simulink model "model_of_system_theta_DC"  (R2021a)
settings: Solver=VariableStepAuto  StartTime=0.0  StopTime=86400  RelTol=1e-3
libraries: fl_lib x88, nesl_utility x28, ee_lib x18, SimscapeFluids_lib x6, simulink x1
(part 1 of 2)
settings Model: OrderedModelArguments=off  Creator=SINA  LastModifiedBy=SINA
settings SolverCC: ZeroCrossAlgorithm=Adaptive
settings DebuggingCC: IgnoredZcDiagnostic=none

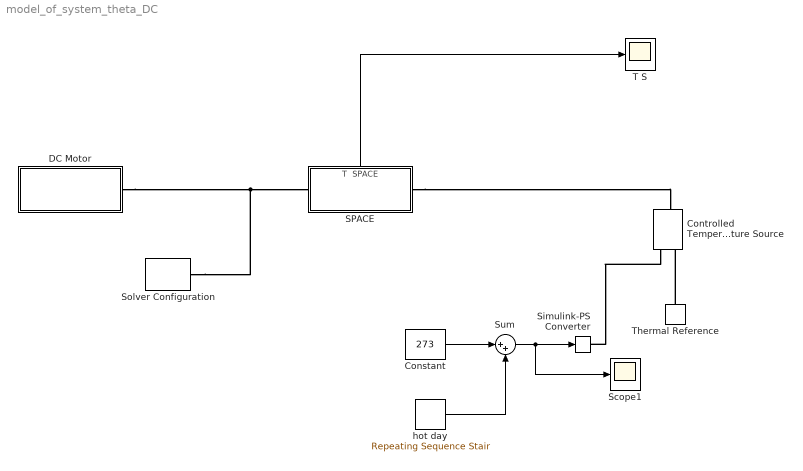
== system model_of_system_theta_DC ==
  Constant : Constant  Value=273
  Controlled Temperature Source : fl_lib/Thermal/Thermal Sources/Controlled Temperature Source
  DC Motor : Subsystem
  "SPACE " : Subsystem
      settings: PortSchema="{\"entries\":[{\"content\":{\"sides\":[{\"content\":{\"connectorIds\":[\"LConn1\"]},\"type\":\"ConnectorPlacement.EquallySpacedRectSide\",\"uuid\":\"d6720360-fd14-4102-8920-24b0f3e87daf\"},{\"content\":{\"connectorIds\":[\"RConn1\"],\"side\":\"RIGHT\"},\"type\":\"ConnectorPlacement.EquallySpacedRectSide\",\"uuid\":\"8de063fd-0e95-49b0-b131-452f09033aa1\"},{\"content\":{\"connectorIds\":[\"Out1\"],\"side\":\"TOP\"},\"type\":\"ConnectorPlacement.EquallySpacedRectSide\",\"uuid\":\"37599775-f873-4ff0-934d-fcf325c50c65\"}]},\"type\":\"ConnectorPlacement.EquallySpacedConnector\",\"uuid\":\"8fae0317-fc8f-430a-90e7-4ae7dd04f39d\"}],\"packageUris\":[\"http://schema.mathworks.com/mf0/Connector/R2020b\"],\"version\":\"1.0\"}"
  Scope1 : Scope
  Simulink-PS Converter : nesl_utility/Simulink-PS Converter  PhysicalDomain=network_engine_domain  SubClassName=ps_input  LeftPortType=input  RightPortType=output  PseudoPeriodic=off  Frequencies=[]  NoiseDistribution=none  NoiseParameters=[]  Unit=K  AffineConversion=off  FilteringAndDerivatives=provide  SimscapeFilterOrder=1  InputFilterTimeConstant=0.001  UdotUserProvided=0
      settings: SourceProductBaseCode=PW,SS
  Solver Configuration : nesl_utility/Solver Configuration  PhysicalDomain=network_engine_domain  SubClassName=solver  LeftPortType=input  RightPortType=generic  Tones=[]  Harmonics=[]  SimulateNoise=off  Profile=off  UseLocalSampling=off  EnableSwitchedLinearOptims=on  FrequencyDomain=off  UseCCode=off  RelTol=0.001  AbsTol=1e-06  MinStep=1e-09  ToWorkspace=off  RevertToSquareIcSolve=off  NumHomotopyIterations=100  PhasorMode=off  PhasorModeNumHarmonics=1  DoDC=off  ResidualTolerance=1e-09  UseLocalSolver=off  LocalSolverChoice=NE_BACKWARD_EULER_ADVANCER  LocalSolverSampleTime=0.001  DoFixedCost=off  MaxNonlinIter=3  MaxModeIter=2  ComputeImpulses=off  ImpulseIterations=2  LinearAlgebra=auto  EquationFormulation=NE_TIME_EF  DelaysMemoryBudget=1024  AutomaticFiltering=on  FilteringTimeConstant=0.001  PartitionStorageMethod=AS_NEEDED  PartitionMemoryBudget=1024  PartitionMethod=ROBUST
      settings: SourceProductBaseCode=PW,SS
  Sum : Sum  Inputs=|++
  T S : Scope
  Thermal Reference : fl_lib/Thermal/Thermal Elements/Thermal Reference
  "hot day " : simulink/Sources/Repeating Sequence Stair  OutValues=|  tsamp=600  OutMin=[]  OutMax=[]  OutDataTypeStr=double  OutputDataTypeScalingMode=double  OutDataType=fixdt(0,8)  ConRadixGroup=Best Precision: Vector-wise  OutScaling=2^-12
      | [19.7
      | 19.8
      | 19.9
      | 19.6
      | 19.3
      | 19
      | 18.9
      | 18.8
      | 18.7
      | 18.6
      | 18.4
      | 18.3
      | 18.4
      | 18.5
      | 18.6
      | 18.6
      | 18.7
      | 18.5
      | 18.5
      | 18.5
      | 18.7
      | 18.9
      | 19.1
      | 19.6
      | 20
      | 20.3
      | 20.7
      | 20.9
      | 20.8
      | 20.7
      | 20.8
      | 21.4
      | 22.1
      | 22.7
      | 23
      | 23.7
      | 24.3
      | 25.2
      | 25.8
      | 25.8
      | 26.2
      | 26.5
      | 26.7
      | 26.7
      | 26.7
      | 27.8
      | 28.2
      | 28.4
      | 29.1
      | 29.5
      | 30.2
      | 30.8
      | 30.8
      | 31.2
      | 31.5
      | 31.4
      | 31.3
      | 31.3
      | 31.2
      | 31.4
      | 31.5
      | 31.5
      | 31.6
      | 31.5
      | 31.6
      | 31.3
      | 31.2
      | 31.2
      | 31.2
      | 31.9
      | 31.7
      | 31.4
      | 31.3
      | 31.6
      | 32.4
      | 32.3
      | 31.9
      | 32
      | 32.1
      | 32.1
      | 32.2
      | 32
      | 32.1
      | 32.1
      | 32.3
      | 32.3
      | 31.9
      | 31.4
      | 31.5
      | 31.5
      | 31
      | 30.6
      | 29.7
      | 28.9
      | 28.4
      | 28.1
      | 27.4
      | 26.6
      | 25.6
      | 24.5
      | 23.7
      | 22.9
      | 22.5
      | 22.2
      | 22
      | 21.9
      | 21.7
      | 21.4
      | 21.2
      | 21.1
      | 20.9
      | 20.9
      | 20.8
      | 20.7
      | 20.6
      | 20.2
      | 20
      | 19.9
      | 19.9
      | 19.9
      | 19.8
      | 19.6
      | 19.4
      | 19.1
      | 19
      | 19
      | 19
      | 18.9
      | 18.8
      | 18.7
      | 18.7
      | 18.3
      | 18
      | 17.7
      | 17.5
      | 17.5
      | 17.4
      | 17.3
      | 17.1
      | 17
      | 16.9
      | 16.8
      | 16.6
      | 16.5
      | 16.5
      | ]
  wires:
  Constant/1 -> Sum/1
  Sum/1 -> Scope1/1, Simulink-PS Converter/1
  "hot day "/1 -> Sum/2
  "SPACE "/1(T  SPACE) -> T S/1
  connections:
  Thermal Reference/LConn1 -- Controlled Temperature Source/RConn2
  Controlled Temperature Source/RConn1 -- Simulink-PS Converter/RConn1
  "SPACE "/RConn1 -- Controlled Temperature Source/LConn1
  DC Motor/LConn1 -- Solver Configuration/RConn1 -- "SPACE "/LConn1

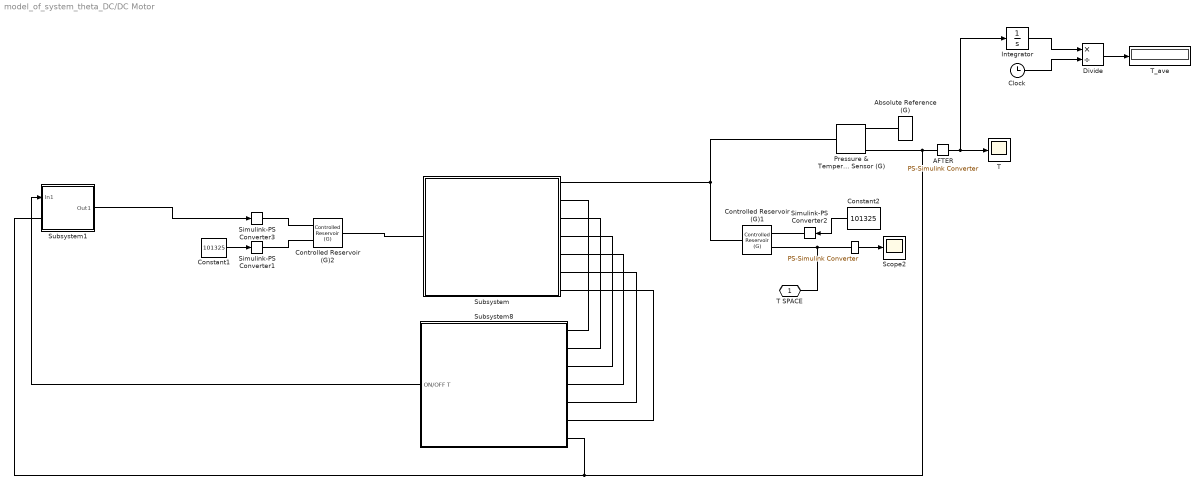
== system model_of_system_theta_DC/DC Motor ==
  " " : nesl_utility/PS-Simulink Converter  PhysicalDomain=network_engine_domain  SubClassName=ps_output  LeftPortType=input  RightPortType=output  PseudoPeriodic=off  Frequencies=[]  Unit=K  AffineConversion=off
      settings: SourceProductBaseCode=PW,SS
  AFTER : nesl_utility/PS-Simulink Converter  PhysicalDomain=network_engine_domain  SubClassName=ps_output  LeftPortType=input  RightPortType=output  PseudoPeriodic=off  Frequencies=[]  Unit=K  AffineConversion=off
      settings: SourceProductBaseCode=PW,SS
  Absolute Reference (G) : fl_lib/Gas/Elements/Absolute Reference (G)
      settings: SourceProductBaseCode=SS  InternalSimscapePortConfiguration="{\"Bottom\":[],\"Left\":[{\"id\":\"A\",\"label\":\"\",\"type\":\"foundation.gas.gas\"}],\"Right\":[],\"Top\":[]}"
  Clock : Clock
  Constant1 : Constant  Value=101325
  Constant2 : Constant  Value=101325
  Controlled Reservoir (G)1 : fl_lib/Gas/Elements/Controlled Reservoir (G)  area_A=25 m^2
      settings: SourceProductBaseCode=SS  InternalSimscapePortConfiguration="{\"Bottom\":[],\"Left\":[{\"id\":\"A\",\"label\":\"A\",\"type\":\"foundation.gas.gas\"}],\"Right\":[{\"id\":\"T_in\",\"label\":\"T\",\"type\":\"input\"},{\"id\":\"p_in\",\"label\":\"P\",\"type\":\"input\"}],\"Top\":[]}"
  Controlled Reservoir (G)2 : fl_lib/Gas/Elements/Controlled Reservoir (G)  area_A=40 m^2
      settings: SourceProductBaseCode=SS  InternalSimscapePortConfiguration="{\"Bottom\":[],\"Left\":[{\"id\":\"A\",\"label\":\"A\",\"type\":\"foundation.gas.gas\"}],\"Right\":[{\"id\":\"T_in\",\"label\":\"T\",\"type\":\"input\"},{\"id\":\"p_in\",\"label\":\"P\",\"type\":\"input\"}],\"Top\":[]}"
  Divide : Product  Inputs=*/
  Integrator : Integrator
  Pressure & Temperature Sensor (G) : fl_lib/Gas/Sensors/Pressure & Temperature Sensor (G)
      settings: SourceProductBaseCode=SS  InternalSimscapePortConfiguration="{\"Bottom\":[],\"Left\":[{\"id\":\"A\",\"label\":\"A\",\"type\":\"foundation.gas.gas\"}],\"Right\":[{\"id\":\"B\",\"label\":\"B\",\"type\":\"foundation.gas.gas\"},{\"id\":\"P\",\"label\":\"P\",\"type\":\"output\"},{\"id\":\"T\",\"label\":\"T\",\"type\":\"output\"}],\"Top\":[]}"
  Scope2 : Scope
  Simulink-PS Converter1 : nesl_utility/Simulink-PS Converter  PhysicalDomain=network_engine_domain  SubClassName=ps_input  LeftPortType=input  RightPortType=output  PseudoPeriodic=off  Frequencies=[]  NoiseDistribution=none  NoiseParameters=[]  Unit=Pa  AffineConversion=off  FilteringAndDerivatives=provide  SimscapeFilterOrder=1  InputFilterTimeConstant=0.001  UdotUserProvided=0
      settings: SourceProductBaseCode=PW,SS
  Simulink-PS Converter2 : nesl_utility/Simulink-PS Converter  PhysicalDomain=network_engine_domain  SubClassName=ps_input  LeftPortType=input  RightPortType=output  PseudoPeriodic=off  Frequencies=[]  NoiseDistribution=none  NoiseParameters=[]  Unit=Pa  AffineConversion=off  FilteringAndDerivatives=provide  SimscapeFilterOrder=1  InputFilterTimeConstant=0.001  UdotUserProvided=0
      settings: SourceProductBaseCode=PW,SS
  Simulink-PS Converter3 : nesl_utility/Simulink-PS Converter  PhysicalDomain=network_engine_domain  SubClassName=ps_input  LeftPortType=input  RightPortType=output  PseudoPeriodic=off  Frequencies=[]  NoiseDistribution=none  NoiseParameters=[]  Unit=K  AffineConversion=off  FilteringAndDerivatives=provide  SimscapeFilterOrder=1  InputFilterTimeConstant=0.001  UdotUserProvided=0
      settings: SourceProductBaseCode=PW,SS
  Subsystem : Subsystem
  Subsystem1 : Subsystem
  Subsystem8 : Subsystem
  T : Scope
  T_ave : Display
  "T SPACE " : PMIOPort  Side=Left
  wires:
  Constant1/1 -> Simulink-PS Converter1/1
  " "/1 -> Scope2/1
  Constant2/1 -> Simulink-PS Converter2/1
  Clock/1 -> Divide/2
  Divide/1 -> T_ave/1
  Integrator/1 -> Divide/1
  AFTER/1 -> T/1, Integrator/1
  Subsystem8/1(ON/OFF T) -> Subsystem1/1(In1)
  Subsystem1/1(Out1) -> Simulink-PS Converter3/1
  connections:
  " "/LConn1 -- "T SPACE "/RConn1 -- Controlled Reservoir (G)1/RConn1
  Simulink-PS Converter3/RConn1 -- Controlled Reservoir (G)2/RConn1
  Simulink-PS Converter1/RConn1 -- Controlled Reservoir (G)2/RConn2
  Simulink-PS Converter2/RConn1 -- Controlled Reservoir (G)1/RConn2
  Absolute Reference (G)/LConn1 -- Pressure & Temperature Sensor (G)/RConn1
  Pressure & Temperature Sensor (G)/LConn1 -- Controlled Reservoir (G)1/LConn1 -- Subsystem/RConn1
  Subsystem/LConn1 -- Controlled Reservoir (G)2/LConn1
  Subsystem8/LConn1 -- Subsystem/RConn2
  Subsystem8/LConn2 -- Subsystem/RConn3
  Subsystem8/LConn3 -- Subsystem/RConn4
  Subsystem8/LConn4 -- Subsystem/RConn5
  Subsystem8/LConn5 -- Subsystem/RConn6
  Subsystem/RConn7 -- Subsystem8/LConn6
  AFTER/LConn1 -- Subsystem1/LConn1 -- Subsystem8/LConn7 -- Pressure & Temperature Sensor (G)/RConn3

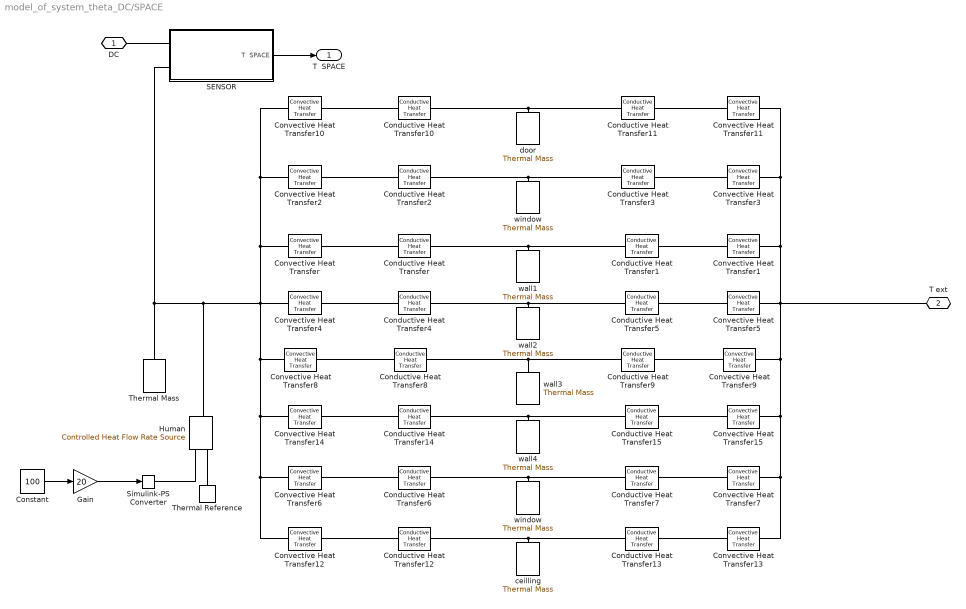
== system model_of_system_theta_DC/SPACE  ==
  " ceilling" : fl_lib/Thermal/Thermal Elements/Thermal Mass  mass=6400 kg  sp_heat=835 J/kg/K  T_specify=on  T_priority=None  T=295 K  T_nominal_specify=off  T_nominal_unit=K  T_nominal_value=1  Q_specify=off  Q_priority=None  Q=0 W  Q_nominal_specify=off  Q_nominal_unit=W  Q_nominal_value=1
  " window" : fl_lib/Thermal/Thermal Elements/Thermal Mass  mass=162 kg  sp_heat=840 J/kg/K  T_specify=on  T_priority=None  T=295 K  T_nominal_specify=off  T_nominal_unit=K  T_nominal_value=1  Q_specify=off  Q_priority=None  Q=0 W  Q_nominal_specify=off  Q_nominal_unit=W  Q_nominal_value=1
  Conductive Heat Transfer{,1,4..5} (4 alike) : fl_lib/Thermal/Thermal Elements/Conductive Heat Transfer  area=320 m^2  thickness=.2 m  th_cond=.038 W/(m*K)  T_specify=off  T_priority=None  T=0 K  T_nominal_specify=off  T_nominal_unit=K  T_nominal_value=1  Q_specify=off  Q_priority=None  Q=0 W  Q_nominal_specify=off  Q_nominal_unit=W  Q_nominal_value=1
  Conductive Heat Transfer10 : fl_lib/Thermal/Thermal Elements/Conductive Heat Transfer  area=7 m^2  thickness=0.04 m  th_cond=.78 W/(m*K)  T_specify=off  T_priority=None  T=0 K  T_nominal_specify=off  T_nominal_unit=K  T_nominal_value=1  Q_specify=off  Q_priority=None  Q=0 W  Q_nominal_specify=off  Q_nominal_unit=W  Q_nominal_value=1
  Conductive Heat Transfer11 : fl_lib/Thermal/Thermal Elements/Conductive Heat Transfer  area=7 m^2  thickness=.04 m  th_cond=.78 W/(m*K)  T_specify=off  T_priority=None  T=0 K  T_nominal_specify=off  T_nominal_unit=K  T_nominal_value=1  Q_specify=off  Q_priority=None  Q=0 W  Q_nominal_specify=off  Q_nominal_unit=W  Q_nominal_value=1
  Conductive Heat Transfer12 : fl_lib/Thermal/Thermal Elements/Conductive Heat Transfer  area=1000 m^2  thickness=0.1 m  th_cond=.038 W/(m*K)  T_specify=off  T_priority=None  T=0 K  T_nominal_specify=off  T_nominal_unit=K  T_nominal_value=1  Q_specify=off  Q_priority=None  Q=0 W  Q_nominal_specify=off  Q_nominal_unit=W  Q_nominal_value=1
  Conductive Heat Transfer13 : fl_lib/Thermal/Thermal Elements/Conductive Heat Transfer  area=1e-4 m^2  thickness=0.1 m  th_cond=.038 W/(m*K)  T_specify=off  T_priority=None  T=0 K  T_nominal_specify=off  T_nominal_unit=K  T_nominal_value=1  Q_specify=off  Q_priority=None  Q=0 W  Q_nominal_specify=off  Q_nominal_unit=W  Q_nominal_value=1
  Conductive Heat Transfer{8..9,14..15} (4 alike) : fl_lib/Thermal/Thermal Elements/Conductive Heat Transfer  area=150 m^2  thickness=.2 m  th_cond=.038 W/(m*K)  T_specify=off  T_priority=None  T=0 K  T_nominal_specify=off  T_nominal_unit=K  T_nominal_value=1  Q_specify=off  Q_priority=None  Q=0 W  Q_nominal_specify=off  Q_nominal_unit=W  Q_nominal_value=1
  Conductive Heat Transfer{2..3,6..7} (4 alike) : fl_lib/Thermal/Thermal Elements/Conductive Heat Transfer  area=6 m^2  thickness=.01 m  th_cond=.78 W/(m*K)  T_specify=off  T_priority=None  T=0 K  T_nominal_specify=off  T_nominal_unit=K  T_nominal_value=1  Q_specify=off  Q_priority=None  Q=0 W  Q_nominal_specify=off  Q_nominal_unit=W  Q_nominal_value=1
  Constant : Constant  Value=100
  Convective Heat Transfer{,1,4..5} (4 alike) : fl_lib/Thermal/Thermal Elements/Convective Heat Transfer  area=320 m^2  heat_tr_coeff=24 W/(m^2 * K)  T_specify=off  T_priority=None  T=0 K  T_nominal_specify=off  T_nominal_unit=K  T_nominal_value=1  Q_specify=off  Q_priority=None  Q=0 W  Q_nominal_specify=off  Q_nominal_unit=W  Q_nominal_value=1
  Convective Heat Transfer10 : fl_lib/Thermal/Thermal Elements/Convective Heat Transfer  area=7 m^2  heat_tr_coeff=26 W/(m^2 * K)  T_specify=off  T_priority=None  T=0 K  T_nominal_specify=off  T_nominal_unit=K  T_nominal_value=1  Q_specify=off  Q_priority=None  Q=0 W  Q_nominal_specify=off  Q_nominal_unit=W  Q_nominal_value=1
  Convective Heat Transfer11 : fl_lib/Thermal/Thermal Elements/Convective Heat Transfer  area=7 m^2  heat_tr_coeff=26 W/(m^2 * K)  T_specify=off  T_priority=None  T=0 K  T_nominal_specify=off  T_nominal_unit=K  T_nominal_value=1  Q_specify=off  Q_priority=None  Q=0 W  Q_nominal_specify=off  Q_nominal_unit=W  Q_nominal_value=1
  Convective Heat Transfer12 : fl_lib/Thermal/Thermal Elements/Convective Heat Transfer  area=1000 m^2  heat_tr_coeff=12 W/(m^2 * K)  T_specify=off  T_priority=None  T=0 K  T_nominal_specify=off  T_nominal_unit=K  T_nominal_value=1  Q_specify=off  Q_priority=None  Q=0 W  Q_nominal_specify=off  Q_nominal_unit=W  Q_nominal_value=1
  Convective Heat Transfer13 : fl_lib/Thermal/Thermal Elements/Convective Heat Transfer  area=1000 m^2  heat_tr_coeff=12 W/(m^2 * K)  T_specify=off  T_priority=None  T=0 K  T_nominal_specify=off  T_nominal_unit=K  T_nominal_value=1  Q_specify=off  Q_priority=None  Q=0 W  Q_nominal_specify=off  Q_nominal_unit=W  Q_nominal_value=1
  Convective Heat Transfer{8..9,14..15} (4 alike) : fl_lib/Thermal/Thermal Elements/Convective Heat Transfer  area=150 m^2  heat_tr_coeff=24 W/(m^2 * K)  T_specify=off  T_priority=None  T=0 K  T_nominal_specify=off  T_nominal_unit=K  T_nominal_value=1  Q_specify=off  Q_priority=None  Q=0 W  Q_nominal_specify=off  Q_nominal_unit=W  Q_nominal_value=1
  Convective Heat Transfer{2..3,6..7} (4 alike) : fl_lib/Thermal/Thermal Elements/Convective Heat Transfer  area=6 m^2  heat_tr_coeff=25 W/(m^2 * K)  T_specify=off  T_priority=None  T=0 K  T_nominal_specify=off  T_nominal_unit=K  T_nominal_value=1  Q_specify=off  Q_priority=None  Q=0 W  Q_nominal_specify=off  Q_nominal_unit=W  Q_nominal_value=1
  Gain : Gain  Gain=20
  Human : fl_lib/Thermal/Thermal Sources/Controlled Heat Flow Rate Source
  SENSOR : Subsystem
  Simulink-PS Converter : nesl_utility/Simulink-PS Converter  PhysicalDomain=network_engine_domain  SubClassName=ps_input  LeftPortType=input  RightPortType=output  PseudoPeriodic=off  Frequencies=[]  NoiseDistribution=none  NoiseParameters=[]  Unit=J/s  AffineConversion=off  FilteringAndDerivatives=provide  SimscapeFilterOrder=1  InputFilterTimeConstant=0.001  UdotUserProvided=0
      settings: SourceProductBaseCode=PW,SS
  Thermal Mass : fl_lib/Thermal/Thermal Elements/Thermal Mass  mass=10200 kg  sp_heat=1 J/kg/K  T_specify=on  T_priority=High  T=295 K  T_nominal_specify=off  T_nominal_unit=K  T_nominal_value=1  Q_specify=off  Q_priority=None  Q=0 W  Q_nominal_specify=off  Q_nominal_unit=W  Q_nominal_value=1
  Thermal Reference : fl_lib/Thermal/Thermal Elements/Thermal Reference
  door : fl_lib/Thermal/Thermal Elements/Thermal Mass  mass=165 kg  sp_heat=840 J/kg/K  T_specify=on  T_priority=None  T=295 K  T_nominal_specify=off  T_nominal_unit=K  T_nominal_value=1  Q_specify=off  Q_priority=None  Q=0 W  Q_nominal_specify=off  Q_nominal_unit=W  Q_nominal_value=1
  wall1 : fl_lib/Thermal/Thermal Elements/Thermal Mass  mass=122880 kg  sp_heat=835 J/kg/K  T_specify=on  T_priority=None  T=295 K  T_nominal_specify=off  T_nominal_unit=K  T_nominal_value=1  Q_specify=off  Q_priority=None  Q=0 W  Q_nominal_specify=off  Q_nominal_unit=W  Q_nominal_value=1
  wall2 : fl_lib/Thermal/Thermal Elements/Thermal Mass  mass=122880 kg  sp_heat=835 J/kg/K  T_specify=on  T_priority=None  T=295 K  T_nominal_specify=off  T_nominal_unit=K  T_nominal_value=1  Q_specify=off  Q_priority=None  Q=0 W  Q_nominal_specify=off  Q_nominal_unit=W  Q_nominal_value=1
  wall3 : fl_lib/Thermal/Thermal Elements/Thermal Mass  mass=57600 kg  sp_heat=835 J/kg/K  T_specify=on  T_priority=None  T=295 K  T_nominal_specify=off  T_nominal_unit=K  T_nominal_value=1  Q_specify=off  Q_priority=None  Q=0 W  Q_nominal_specify=off  Q_nominal_unit=W  Q_nominal_value=1
  wall4 : fl_lib/Thermal/Thermal Elements/Thermal Mass  mass=57600 kg  sp_heat=835 J/kg/K  T_specify=on  T_priority=None  T=295 K  T_nominal_specify=off  T_nominal_unit=K  T_nominal_value=1  Q_specify=off  Q_priority=None  Q=0 W  Q_nominal_specify=off  Q_nominal_unit=W  Q_nominal_value=1
  window : fl_lib/Thermal/Thermal Elements/Thermal Mass  mass=162 kg  sp_heat=840 J/kg/K  T_specify=on  T_priority=None  T=295 K  T_nominal_specify=off  T_nominal_unit=K  T_nominal_value=1  Q_specify=off  Q_priority=None  Q=0 W  Q_nominal_specify=off  Q_nominal_unit=W  Q_nominal_value=1
  DC : PMIOPort  Side=Left
  T ext : PMIOPort  Port=2  Side=Right
  T  SPACE : Outport  SampleTime=1
  wires:
  SENSOR/1(T  SPACE) -> T  SPACE/1
  Constant/1 -> Gain/1
  Gain/1 -> Simulink-PS Converter/1
  connections:
  Convective Heat Transfer/RConn1 -- Conductive Heat Transfer/LConn1
  Conductive Heat Transfer/RConn1 -- Conductive Heat Transfer1/LConn1 -- wall1/LConn1
  Convective Heat Transfer1/LConn1 -- Conductive Heat Transfer1/RConn1
  Conductive Heat Transfer3/LConn1 -- Conductive Heat Transfer2/RConn1 -- window/LConn1
  Convective Heat Transfer2/RConn1 -- Conductive Heat Transfer2/LConn1
  Convective Heat Transfer3/LConn1 -- Conductive Heat Transfer3/RConn1
  Conductive Heat Transfer5/LConn1 -- Conductive Heat Transfer4/RConn1 -- wall2/LConn1
  Convective Heat Transfer4/RConn1 -- Conductive Heat Transfer4/LConn1
  Convective Heat Transfer5/LConn1 -- Conductive Heat Transfer5/RConn1
  Conductive Heat Transfer6/RConn1 -- Conductive Heat Transfer7/LConn1 -- " window"/LConn1
  Convective Heat Transfer7/LConn1 -- Conductive Heat Transfer7/RConn1
  Convective Heat Transfer6/RConn1 -- Conductive Heat Transfer6/LConn1
  Convective Heat Transfer2/LConn1 -- Convective Heat Transfer10/LConn1 -- Human/LConn1 -- SENSOR/LConn2 -- Thermal Mass/LConn1 -- Convective Heat Transfer4/LConn1 -- Convective Heat Transfer14/LConn1 -- Convective Heat Transfer12/LConn1 -- Convective Heat Transfer6/LConn1 -- Convective Heat Transfer8/LConn1 -- Convective Heat Transfer/LConn1
  Conductive Heat Transfer8/RConn1 -- Conductive Heat Transfer9/LConn1 -- wall3/LConn1
  Convective Heat Transfer9/LConn1 -- Conductive Heat Transfer9/RConn1
  Convective Heat Transfer8/RConn1 -- Conductive Heat Transfer8/LConn1
  Conductive Heat Transfer10/RConn1 -- Conductive Heat Transfer11/LConn1 -- door/LConn1
  Convective Heat Transfer11/LConn1 -- Conductive Heat Transfer11/RConn1
  Convective Heat Transfer10/RConn1 -- Conductive Heat Transfer10/LConn1
  Convective Heat Transfer11/RConn1 -- Convective Heat Transfer5/RConn1 -- Convective Heat Transfer15/RConn1 -- Convective Heat Transfer13/RConn1 -- Convective Heat Transfer7/RConn1 -- Convective Heat Transfer9/RConn1 -- T ext/RConn1 -- Convective Heat Transfer1/RConn1 -- Convective Heat Transfer3/RConn1
  Conductive Heat Transfer13/LConn1 -- " ceilling"/LConn1 -- Conductive Heat Transfer12/RConn1
  Convective Heat Transfer13/LConn1 -- Conductive Heat Transfer13/RConn1
  Convective Heat Transfer12/RConn1 -- Conductive Heat Transfer12/LConn1
  DC/RConn1 -- SENSOR/LConn1
  Conductive Heat Transfer14/RConn1 -- Conductive Heat Transfer15/LConn1 -- wall4/LConn1
  Convective Heat Transfer15/LConn1 -- Conductive Heat Transfer15/RConn1
  Convective Heat Transfer14/RConn1 -- Conductive Heat Transfer14/LConn1
  Human/RConn1 -- Simulink-PS Converter/RConn1
  Thermal Reference/LConn1 -- Human/RConn2

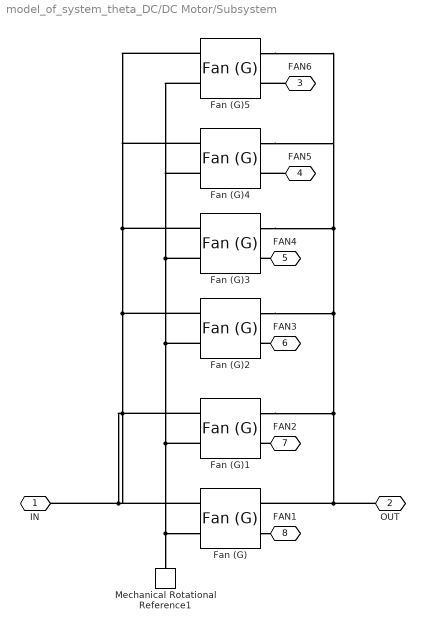
== system model_of_system_theta_DC/DC Motor/Subsystem ==
  Fan (G){,1..4} (5 alike) : SimscapeFluids_lib/Gas/Turbomachinery/Fan (G)  fan_spec=fluids.gas.enum.fan_spec.table2D_dp_dpmax_omega  mech_orientation=simscape.enum.posneg.positive  flow_rate_1D_TLU=[4.7, 5.2, 5.7, 6.1, 6.6] m^3/s  Dp_1D_TLU=[1120, 995.36, 870.94, 746.52, 622.1] Pa  eta_1D_TLU=[.1, .2, .25, .15, .1]  rho_ref_1D=1.2 kg/m^3  omega_ref_1D=910 rpm  omega_Dp_TLU=[2000,2500,3000] rpm  flow_rate_Dp_TLU=[.2, .3, .4, .5] m^3/s  Dp_TLU=[675, 650, 560, 420; 830, 800, 695, 520; 1008, 966, 840, 630; 1200, 1150, 1000, 750; 1370, 1300, 1250, 1000] Pa  eta_Dp_TLU=ones(3,20).*0.3  omega_flow_TLU=[1800, 2000, 2400, 2800, 3000] rpm  Dp_flow_TLU=[1 / 8, 1 / 4, 3 / 8, 1 / 2] * 3386.4 Pa  flow_rate_TLU=[.3282, .2965, .2556, .1973; .8254, .71, .5876, .4545; 1.2018, 1.0829, .9083, .7034; 1.5065, 1.4098, 1.2722, .9844; 1.8368, 1.7507, 1.6055, 1.2417] m^3/s  eta_flow_TLU=[.22, .23, .25, .24; .38, .39, .4, .34; .58, .6, .62, .6; .81, .82, .84, .8; .88, .91, .95, .9]  omega_DpMax_TLU=[2000,2500,3000] rpm  DpMax_TLU=[16.100000000000000,24.500000000000000,34.800000000000000] Pa  omega_flow_TLU_=[2000,2500,3000] rpm  Dp_DpMax_TLU=[0,0.0526315789473684,0.105263157894737,0.157894736842105,0.210526315789474,0.263157894736842,0.315789473684211,0.368421052631579,0.421052631578947,0.473684210526316,0.526315789473684,0.578947368421053,0.631578947368421,0.684210526315790,0.736842105263158,0.789473684210526,0.842105263157895,0.894736842105263,0.947368421052632,1]  flow_rate_TLU_=[16.1273000000000,15.8178000000000,15.0681000000000,14.2018000000000,12.9433000000000,11.3991000000000,9.67790000000000,8.08610000000000,7.01870000000000,6.30920000000000,5.93980000000000,5.97320000000000,5.86980000000000,5.71970000000000,5.52780000000000,5.20060000000000,4.55740000000000,3.42180000000000,1.76410000000000,0.000100000000000000;24.5333000000000,24.3970000000000,23.8165000000000,23.1737000000000,21.5953000000000,19.0999000000000,16.6546000000000,14.3745000000000,12.7327000000000,11.8387000000000,11.3795000000000,11.0625000000000,10.7728000000000,10.4860000000000,10.0474000000000,9.13940000000000,7.85700000000000,5.63250000000000,3.16660000000000,0.000100000000000000;34.8365000000000,34.2986000000000,33.4330000000000,32.3142000000000,30.4522000000000,27.7361000000000,24.3880000000000,21.6723000000000,19.7551000000000,18.4534000000000,17.3506000000000,16.6400000000000,15.8701000000000,14.8205000000000,13.6975000000000,11.7356000000000,9.67960000000000,6.82460000000000,3.51230000000000,0.000100000000000000] lpm  eta_flow_TLU_=ones(3,20).*0.3  rho_ref_2D=1.2 kg/m^3  omega_threshold=1 rpm  area_A=2 m^2  area_B=2 m^2
      settings: SourceProductBaseCode=SH  InternalSimscapePortConfiguration="{\"Bottom\":[],\"Left\":[{\"id\":\"A\",\"label\":\"A\",\"type\":\"foundation.gas.gas\"},{\"id\":\"C\",\"label\":\"C\",\"type\":\"foundation.mechanical.rotational.rotational\"}],\"Right\":[{\"id\":\"B\",\"label\":\"B\",\"type\":\"foundation.gas.gas\"},{\"id\":\"R\",\"label\":\"R\",\"type\":\"foundation.mechanical.rotational.rotational\"}],\"Top\":[]}"
  Fan (G)5 : SimscapeFluids_lib/Gas/Turbomachinery/Fan (G)  fan_spec=fluids.gas.enum.fan_spec.table2D_dp_dpmax_omega  mech_orientation=simscape.enum.posneg.positive  flow_rate_1D_TLU=[4.7, 5.2, 5.7, 6.1, 6.6] m^3/s  Dp_1D_TLU=[1120, 995.36, 870.94, 746.52, 622.1] Pa  eta_1D_TLU=[.1, .2, .25, .15, .1]  rho_ref_1D=1.2 kg/m^3  omega_ref_1D=910 rpm  omega_Dp_TLU=[2000,2500,3000] rpm  flow_rate_Dp_TLU=[.2, .3, .4, .5] m^3/s  Dp_TLU=[675, 650, 560, 420; 830, 800, 695, 520; 1008, 966, 840, 630; 1200, 1150, 1000, 750; 1370, 1300, 1250, 1000] Pa  eta_Dp_TLU=ones(3,20).*0.3  omega_flow_TLU=[1800, 2000, 2400, 2800, 3000] rpm  Dp_flow_TLU=[1 / 8, 1 / 4, 3 / 8, 1 / 2] * 3386.4 Pa  flow_rate_TLU=[.3282, .2965, .2556, .1973; .8254, .71, .5876, .4545; 1.2018, 1.0829, .9083, .7034; 1.5065, 1.4098, 1.2722, .9844; 1.8368, 1.7507, 1.6055, 1.2417] m^3/s  eta_flow_TLU=[.22, .23, .25, .24; .38, .39, .4, .34; .58, .6, .62, .6; .81, .82, .84, .8; .88, .91, .95, .9]  omega_DpMax_TLU=[2000,2500,3000] rpm  DpMax_TLU=[16.100000000000000,24.500000000000000,34.800000000000000] Pa  omega_flow_TLU_=[2000,2500,3000] rad/s  Dp_DpMax_TLU=[0,0.0526315789473684,0.105263157894737,0.157894736842105,0.210526315789474,0.263157894736842,0.315789473684211,0.368421052631579,0.421052631578947,0.473684210526316,0.526315789473684,0.578947368421053,0.631578947368421,0.684210526315790,0.736842105263158,0.789473684210526,0.842105263157895,0.894736842105263,0.947368421052632,1]  flow_rate_TLU_=[16.1273000000000,15.8178000000000,15.0681000000000,14.2018000000000,12.9433000000000,11.3991000000000,9.67790000000000,8.08610000000000,7.01870000000000,6.30920000000000,5.93980000000000,5.97320000000000,5.86980000000000,5.71970000000000,5.52780000000000,5.20060000000000,4.55740000000000,3.42180000000000,1.76410000000000,0.000100000000000000;24.5333000000000,24.3970000000000,23.8165000000000,23.1737000000000,21.5953000000000,19.0999000000000,16.6546000000000,14.3745000000000,12.7327000000000,11.8387000000000,11.3795000000000,11.0625000000000,10.7728000000000,10.4860000000000,10.0474000000000,9.13940000000000,7.85700000000000,5.63250000000000,3.16660000000000,0.000100000000000000;34.8365000000000,34.2986000000000,33.4330000000000,32.3142000000000,30.4522000000000,27.7361000000000,24.3880000000000,21.6723000000000,19.7551000000000,18.4534000000000,17.3506000000000,16.6400000000000,15.8701000000000,14.8205000000000,13.6975000000000,11.7356000000000,9.67960000000000,6.82460000000000,3.51230000000000,0.000100000000000000] lpm  eta_flow_TLU_=ones(3,20).*0.3  rho_ref_2D=1.2 kg/m^3  omega_threshold=1 rpm  area_A=2 m^2  area_B=2 m^2
      settings: SourceProductBaseCode=SH  InternalSimscapePortConfiguration="{\"Bottom\":[],\"Left\":[{\"id\":\"A\",\"label\":\"A\",\"type\":\"foundation.gas.gas\"},{\"id\":\"C\",\"label\":\"C\",\"type\":\"foundation.mechanical.rotational.rotational\"}],\"Right\":[{\"id\":\"B\",\"label\":\"B\",\"type\":\"foundation.gas.gas\"},{\"id\":\"R\",\"label\":\"R\",\"type\":\"foundation.mechanical.rotational.rotational\"}],\"Top\":[]}"
  Mechanical Rotational Reference1 : fl_lib/Mechanical/Rotational Elements/Mechanical Rotational Reference
  IN : PMIOPort  Side=Left
  OUT : PMIOPort  Port=2  Side=Right
  FAN6 : PMIOPort  Port=3  Side=Right
  FAN5 : PMIOPort  Port=4  Side=Right
  FAN4 : PMIOPort  Port=5  Side=Right
  FAN3 : PMIOPort  Port=6  Side=Right
  FAN2 : PMIOPort  Port=7  Side=Right
  FAN1 : PMIOPort  Port=8  Side=Right
  connections:
  Fan (G)1/RConn1 -- Fan (G)2/RConn1 -- Fan (G)5/RConn1 -- Fan (G)4/RConn1 -- Fan (G)3/RConn1 -- Fan (G)/RConn1 -- OUT/RConn1
  FAN4/RConn1 -- Fan (G)3/RConn2
  Fan (G)/LConn1 -- Fan (G)5/LConn1 -- Fan (G)4/LConn1 -- Fan (G)3/LConn1 -- Fan (G)2/LConn1 -- Fan (G)1/LConn1 -- IN/RConn1
  Fan (G)5/LConn2 -- Fan (G)4/LConn2 -- Fan (G)3/LConn2 -- Fan (G)2/LConn2 -- Fan (G)1/LConn2 -- Mechanical Rotational Reference1/LConn1 -- Fan (G)/LConn2
  FAN2/RConn1 -- Fan (G)1/RConn2
  FAN5/RConn1 -- Fan (G)4/RConn2
  FAN6/RConn1 -- Fan (G)5/RConn2
  FAN3/RConn1 -- Fan (G)2/RConn2
  Fan (G)/RConn2 -- FAN1/RConn1

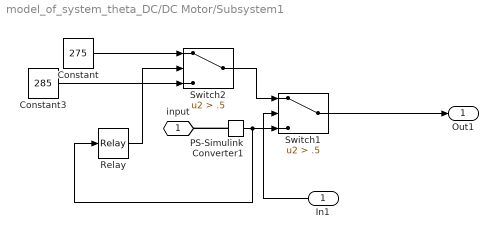
== system model_of_system_theta_DC/DC Motor/Subsystem1 ==
  In1 : Inport
  Constant : Constant  Value=275
  Constant3 : Constant  Value=285
  PS-Simulink Converter1 : nesl_utility/PS-Simulink Converter  PhysicalDomain=network_engine_domain  SubClassName=ps_output  LeftPortType=input  RightPortType=output  PseudoPeriodic=off  Frequencies=[]  Unit=inherit  AffineConversion=off
      settings: SourceProductBaseCode=PW,SS
  Relay : Relay  OnSwitchValue=299  OffSwitchValue=296
  Switch1 : Switch  Criteria=u2 > Threshold  Threshold=.5
  Switch2 : Switch  Criteria=u2 > Threshold  Threshold=.5
  input : PMIOPort  Side=Left
  Out1 : Outport
  wires:
  In1/1 -> Switch1/2
  Switch2/1 -> Switch1/1
  PS-Simulink Converter1/1 -> Relay/1, Switch1/3
  Relay/1 -> Switch2/2
  Constant/1 -> Switch2/1
  Constant3/1 -> Switch2/3
  Switch1/1 -> Out1/1
  connections:
  PS-Simulink Converter1/LConn1 -- input/RConn1

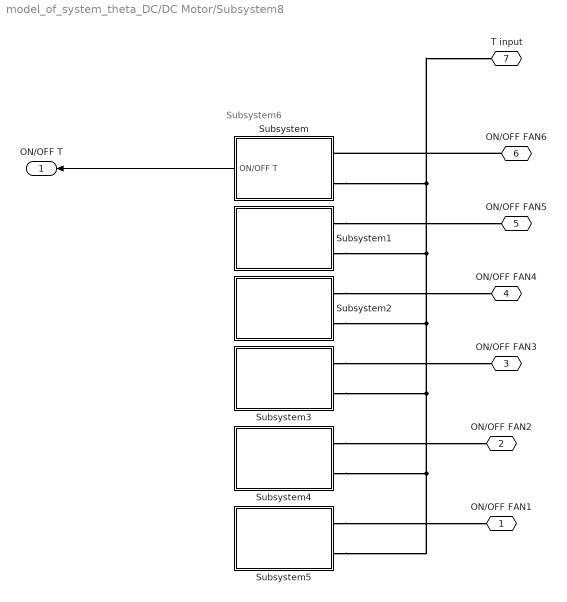
== system model_of_system_theta_DC/DC Motor/Subsystem8 ==
  note: Subsystem6
  Subsystem : Subsystem
  Subsystem1 : Subsystem
  Subsystem2 : Subsystem
  Subsystem3 : Subsystem
  Subsystem4 : Subsystem
  Subsystem5 : Subsystem
  ON/OFF FAN1 : PMIOPort  Side=Left
  ON/OFF FAN2 : PMIOPort  Port=2  Side=Left
  ON/OFF FAN3 : PMIOPort  Port=3  Side=Left
  ON/OFF FAN4 : PMIOPort  Port=4  Side=Left
  ON/OFF FAN5 : PMIOPort  Port=5  Side=Left
  ON/OFF FAN6 : PMIOPort  Port=6  Side=Left
  T input : PMIOPort  Port=7  Side=Left
  ON/OFF T : Outport
  wires:
  Subsystem/1(ON/OFF T) -> ON/OFF T/1
  connections:
  Subsystem1/LConn1 -- ON/OFF FAN5/RConn1
  Subsystem2/LConn1 -- ON/OFF FAN4/RConn1
  Subsystem3/LConn1 -- ON/OFF FAN3/RConn1
  Subsystem4/LConn1 -- ON/OFF FAN2/RConn1
  Subsystem5/LConn1 -- ON/OFF FAN1/RConn1
  Subsystem5/LConn2 -- Subsystem2/LConn2 -- T input/RConn1 -- Subsystem/LConn2 -- Subsystem1/LConn2 -- Subsystem3/LConn2 -- Subsystem4/LConn2
  ON/OFF FAN6/RConn1 -- Subsystem/LConn1

== system model_of_system_theta_DC/SPACE /SENSOR ==
  PS-Simulink Converter : nesl_utility/PS-Simulink Converter  PhysicalDomain=network_engine_domain  SubClassName=ps_output  LeftPortType=input  RightPortType=output  PseudoPeriodic=off  Frequencies=[]  Unit=K  AffineConversion=off
      settings: SourceProductBaseCode=PW,SS
  Scope : Scope
  Temperature Sensor : fl_lib/Thermal/Thermal Sensors/Temperature Sensor
  Thermal Reference1 : fl_lib/Thermal/Thermal Elements/Thermal Reference
  FAN : PMIOPort  Side=Left
  Conn2 : PMIOPort  Port=2  Side=Left
  T  SPACE : Outport  SampleTime=1
  wires:
  PS-Simulink Converter/1 -> T  SPACE/1, Scope/1
  connections:
  Temperature Sensor/RConn2 -- FAN/RConn1 -- PS-Simulink Converter/LConn1
  Temperature Sensor/LConn1 -- Conn2/RConn1
  Thermal Reference1/LConn1 -- Temperature Sensor/RConn1

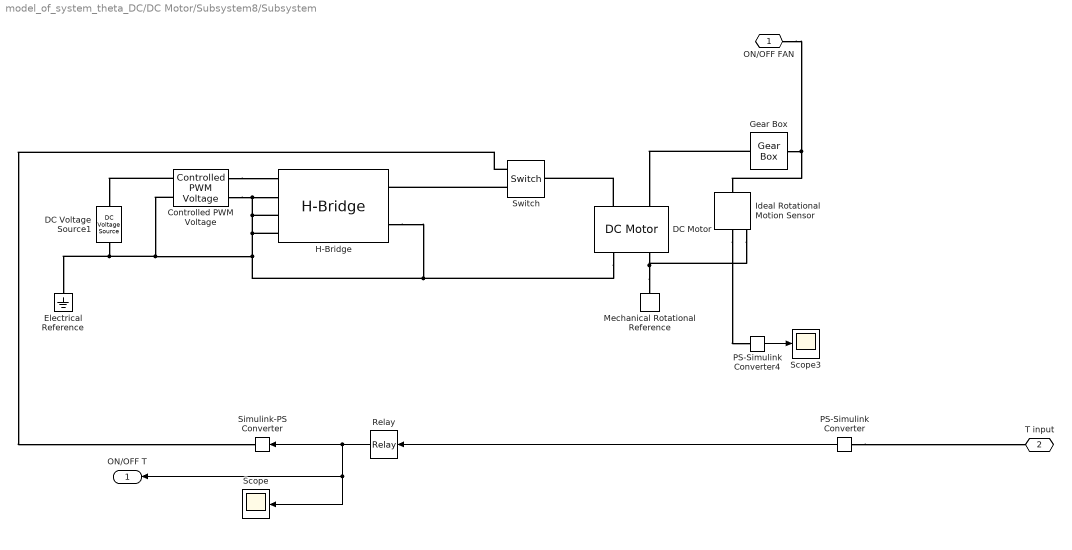
== system model_of_system_theta_DC/DC Motor/Subsystem8/Subsystem ==
  Controlled PWM Voltage : ee_lib/Integrated Circuits/Controlled PWM Voltage  F=4000 Hz  TD=0 s  pulse_width_offset=0 s  pulse_min=0 s  Vmin=0 V  Vmax=5 V  Vm=5 V  pwm_or_av=2  event_type=1  sample_time=1e-6 s  u_min=0  u_max=1
  DC Motor : ee_lib/Electromechanical/Brushed Motors/DC Motor  field_option=ee.enum.field_option.pm  Rf=100 Ohm  Lf=1 H  Laf=0.15 H  If0=0 A  parameterization=ee.enum.dcparam_option.load_speed  Ra=3.9 Ohm  La=.01 H  emf_or_torque=ee.enum.emf_or_torque.kv  Kv=0.072e-3 V/rpm  Ki=6.876e-4 N*m/A  T_stall=0.24e-3 N*m  w_max=4000 rpm  w_rated=1000 rpm  P_rated=10 W  V_rated=12 V  J=0.0002 kg*m^2  lam_param=ee.enum.lam_param.damping  lam=0.5e-5 N*m/(rad/s)  i_noload=0 A  V_i_noload=1.5 V  speed0=0 rpm  enable_fault_armature=ee.enum.faults.faultEnable.no  rev_faulted=1 / 3  G_faulted_armature=1e-5 S  fault_trigger_armature=ee.enum.faults.faultTrigger.temporal  t_fault_armature=1 s  max_permissible_current_armature=inf A  t_fail_on_current_armature=1 s  enable_fault_field=ee.enum.faults.faultEnable.no  G_faulted_field=1e-5 S  fault_trigger_field=ee.enum.faults.faultTrigger.temporal  t_fault_field=1 s  max_permissible_current_field=inf A  t_fail_on_current_field=1 s  fault_action=ee.enum.faults.faultAction.none  alpha=3.93e-3 1/K  Tmeas=25 degC  thermal_mass=100 J/K  initial_temperature=25 degC
  DC Voltage Source1 : fl_lib/Electrical/Electrical Sources/DC Voltage Source  v0=2.5 V
  Electrical Reference : fl_lib/Electrical/Electrical Elements/Electrical Reference
  Gear Box : fl_lib/Mechanical/Mechanisms/Gear Box  ratio=10  t_in_specify=off  t_in_priority=None  t_in=0 N*m  t_in_nominal_specify=off  t_in_nominal_unit=N*m  t_in_nominal_value=1  t_out_specify=off  t_out_priority=None  t_out=0 N*m  t_out_nominal_specify=off  t_out_nominal_unit=N*m  t_out_nominal_value=1
  H-Bridge : ee_lib/Semiconductors & Converters/Converters/H-Bridge  supply_ports=ee.enum.supply_ports.hidesupply  Venable=2.5 V  Vmax=5.0 V  Vreverse=2.5 V  Vbrake=2.5 V  Vm=12 V  pwm_or_av=ee.enum.pwm_or_av.averaged  regenerative_braking_mode=ee.enum.converters.regenerative_braking_mode.depends_on_rev  discontinuous=ee.enum.current_profile.continuous  freewheeling_mode=ee.enum.converters.freewheeling_mode.one_switch_one_diode  Ron=0.1 Ohm  Don=0.05 Ohm  Goff=1e-6 S  Rload=10 Ohm  Lload=1e-5 H  F=10 kHz  thermal_mass=100 J/K  initial_temperature=298.15 K  Ron2=0.1 Ohm  Don2=0.05 Ohm  Tmeas=298.15 K  Tmeas2=398.15 K
  Ideal Rotational Motion Sensor : fl_lib/Mechanical/Mechanical Sensors/Ideal Rotational Motion Sensor  wrap_angle=simscape.enum.onoff.off  offset=0 deg
  Mechanical Rotational Reference : fl_lib/Mechanical/Rotational Elements/Mechanical Rotational Reference
  PS-Simulink Converter : nesl_utility/PS-Simulink Converter  PhysicalDomain=network_engine_domain  SubClassName=ps_output  LeftPortType=input  RightPortType=output  PseudoPeriodic=off  Frequencies=[]  Unit=inherit  AffineConversion=off
      settings: SourceProductBaseCode=PW,SS
  PS-Simulink Converter4 : nesl_utility/PS-Simulink Converter  PhysicalDomain=network_engine_domain  SubClassName=ps_output  LeftPortType=input  RightPortType=output  PseudoPeriodic=off  Frequencies=[]  Unit=rpm  AffineConversion=off
      settings: SourceProductBaseCode=PW,SS
  Relay : Relay  OnSwitchValue=298  OffSwitchValue=295
  Scope : Scope
  Scope3 : Scope
  Simulink-PS Converter : nesl_utility/Simulink-PS Converter  PhysicalDomain=network_engine_domain  SubClassName=ps_input  LeftPortType=input  RightPortType=output  PseudoPeriodic=off  Frequencies=[]  NoiseDistribution=none  NoiseParameters=[]  Unit=1  AffineConversion=off  FilteringAndDerivatives=provide  SimscapeFilterOrder=1  InputFilterTimeConstant=0.001  UdotUserProvided=0
      settings: SourceProductBaseCode=PW,SS
  Switch : fl_lib/Electrical/Electrical Elements/Switch  R_closed=0.01 Ohm  G_open=1e-8 1/Ohm  Threshold=0.5  i_specify=off  i_priority=None  i=0 A  i_nominal_specify=off  i_nominal_unit=A  i_nominal_value=1  v_specify=off  v_priority=None  v=0 V  v_nominal_specify=off  v_nominal_unit=V  v_nominal_value=1
  ON/OFF FAN : PMIOPort  Side=Left
  T input : PMIOPort  Port=2  Side=Left
  ON/OFF T : Outport
  wires:
  Relay/1 -> Scope/1, ON/OFF T/1, Simulink-PS Converter/1
  PS-Simulink Converter4/1 -> Scope3/1
  PS-Simulink Converter/1 -> Relay/1
  connections:
  Switch/RConn1 -- Simulink-PS Converter/RConn1
  DC Voltage Source1/RConn1 -- Controlled PWM Voltage/LConn2 -- H-Bridge/LConn3 -- H-Bridge/LConn2 -- Controlled PWM Voltage/RConn2 -- H-Bridge/LConn4 -- H-Bridge/RConn2 -- DC Motor/RConn1 -- Electrical Reference/LConn1
  Gear Box/LConn1 -- DC Motor/LConn2
  Controlled PWM Voltage/LConn1 -- DC Voltage Source1/LConn1
  Gear Box/RConn1 -- ON/OFF FAN/RConn1 -- Ideal Rotational Motion Sensor/LConn1
  Ideal Rotational Motion Sensor/RConn2 -- PS-Simulink Converter4/LConn1
  Mechanical Rotational Reference/LConn1 -- DC Motor/RConn2 -- Ideal Rotational Motion Sensor/RConn1
  Controlled PWM Voltage/RConn1 -- H-Bridge/LConn1
  Switch/RConn2 -- H-Bridge/RConn1
  DC Motor/LConn1 -- Switch/LConn1
  PS-Simulink Converter/LConn1 -- T input/RConn1

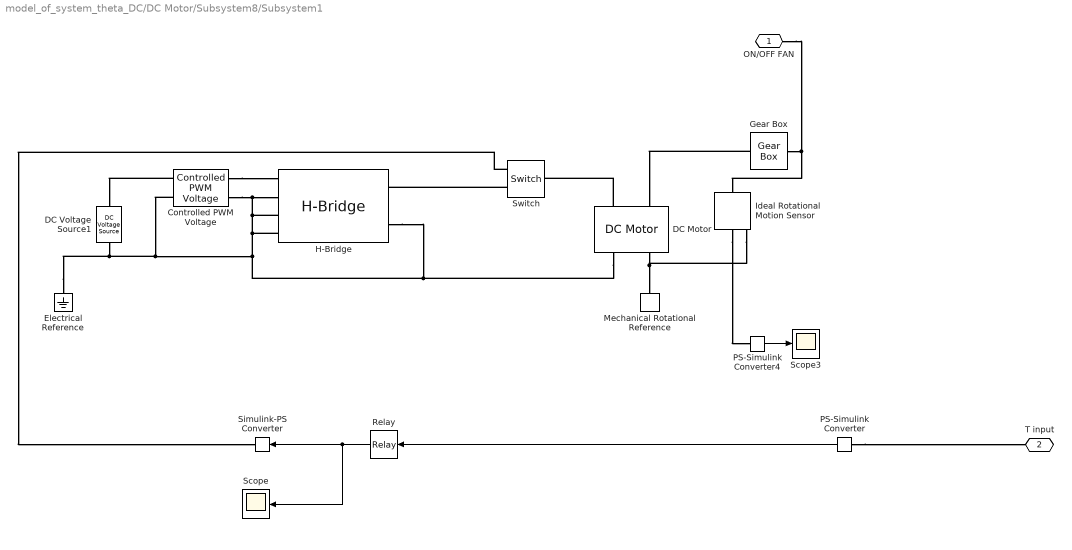
== system model_of_system_theta_DC/DC Motor/Subsystem8/Subsystem1 ==
  Controlled PWM Voltage : ee_lib/Integrated Circuits/Controlled PWM Voltage  F=4000 Hz  TD=0 s  pulse_width_offset=0 s  pulse_min=0 s  Vmin=0 V  Vmax=5 V  Vm=5 V  pwm_or_av=2  event_type=1  sample_time=1e-6 s  u_min=0  u_max=1
  DC Motor : ee_lib/Electromechanical/Brushed Motors/DC Motor  field_option=ee.enum.field_option.pm  Rf=100 Ohm  Lf=1 H  Laf=0.15 H  If0=0 A  parameterization=ee.enum.dcparam_option.load_speed  Ra=3.9 Ohm  La=.01 H  emf_or_torque=ee.enum.emf_or_torque.kv  Kv=0.072e-3 V/rpm  Ki=6.876e-4 N*m/A  T_stall=0.24e-3 N*m  w_max=4000 rpm  w_rated=1000 rpm  P_rated=10 W  V_rated=12 V  J=0.0002 kg*m^2  lam_param=ee.enum.lam_param.damping  lam=0.5e-5 N*m/(rad/s)  i_noload=0 A  V_i_noload=1.5 V  speed0=0 rpm  enable_fault_armature=ee.enum.faults.faultEnable.no  rev_faulted=1 / 3  G_faulted_armature=1e-5 S  fault_trigger_armature=ee.enum.faults.faultTrigger.temporal  t_fault_armature=1 s  max_permissible_current_armature=inf A  t_fail_on_current_armature=1 s  enable_fault_field=ee.enum.faults.faultEnable.no  G_faulted_field=1e-5 S  fault_trigger_field=ee.enum.faults.faultTrigger.temporal  t_fault_field=1 s  max_permissible_current_field=inf A  t_fail_on_current_field=1 s  fault_action=ee.enum.faults.faultAction.none  alpha=3.93e-3 1/K  Tmeas=25 degC  thermal_mass=100 J/K  initial_temperature=25 degC
  DC Voltage Source1 : fl_lib/Electrical/Electrical Sources/DC Voltage Source  v0=2.5 V
  Electrical Reference : fl_lib/Electrical/Electrical Elements/Electrical Reference
  Gear Box : fl_lib/Mechanical/Mechanisms/Gear Box  ratio=10  t_in_specify=off  t_in_priority=None  t_in=0 N*m  t_in_nominal_specify=off  t_in_nominal_unit=N*m  t_in_nominal_value=1  t_out_specify=off  t_out_priority=None  t_out=0 N*m  t_out_nominal_specify=off  t_out_nominal_unit=N*m  t_out_nominal_value=1
  H-Bridge : ee_lib/Semiconductors & Converters/Converters/H-Bridge  supply_ports=ee.enum.supply_ports.hidesupply  Venable=2.5 V  Vmax=5.0 V  Vreverse=2.5 V  Vbrake=2.5 V  Vm=12 V  pwm_or_av=ee.enum.pwm_or_av.averaged  regenerative_braking_mode=ee.enum.converters.regenerative_braking_mode.depends_on_rev  discontinuous=ee.enum.current_profile.continuous  freewheeling_mode=ee.enum.converters.freewheeling_mode.one_switch_one_diode  Ron=0.1 Ohm  Don=0.05 Ohm  Goff=1e-6 S  Rload=10 Ohm  Lload=1e-5 H  F=10 kHz  thermal_mass=100 J/K  initial_temperature=298.15 K  Ron2=0.1 Ohm  Don2=0.05 Ohm  Tmeas=298.15 K  Tmeas2=398.15 K
  Ideal Rotational Motion Sensor : fl_lib/Mechanical/Mechanical Sensors/Ideal Rotational Motion Sensor  wrap_angle=simscape.enum.onoff.off  offset=0 deg
  Mechanical Rotational Reference : fl_lib/Mechanical/Rotational Elements/Mechanical Rotational Reference
  PS-Simulink Converter : nesl_utility/PS-Simulink Converter  PhysicalDomain=network_engine_domain  SubClassName=ps_output  LeftPortType=input  RightPortType=output  PseudoPeriodic=off  Frequencies=[]  Unit=inherit  AffineConversion=off
      settings: SourceProductBaseCode=PW,SS
  PS-Simulink Converter4 : nesl_utility/PS-Simulink Converter  PhysicalDomain=network_engine_domain  SubClassName=ps_output  LeftPortType=input  RightPortType=output  PseudoPeriodic=off  Frequencies=[]  Unit=rpm  AffineConversion=off
      settings: SourceProductBaseCode=PW,SS
  Relay : Relay  OnSwitchValue=298  OffSwitchValue=295
  Scope : Scope
  Scope3 : Scope
  Simulink-PS Converter : nesl_utility/Simulink-PS Converter  PhysicalDomain=network_engine_domain  SubClassName=ps_input  LeftPortType=input  RightPortType=output  PseudoPeriodic=off  Frequencies=[]  NoiseDistribution=none  NoiseParameters=[]  Unit=1  AffineConversion=off  FilteringAndDerivatives=provide  SimscapeFilterOrder=1  InputFilterTimeConstant=0.001  UdotUserProvided=0
      settings: SourceProductBaseCode=PW,SS
  Switch : fl_lib/Electrical/Electrical Elements/Switch  R_closed=0.01 Ohm  G_open=1e-8 1/Ohm  Threshold=0.5  i_specify=off  i_priority=None  i=0 A  i_nominal_specify=off  i_nominal_unit=A  i_nominal_value=1  v_specify=off  v_priority=None  v=0 V  v_nominal_specify=off  v_nominal_unit=V  v_nominal_value=1
  ON/OFF FAN : PMIOPort  Side=Left
  T input : PMIOPort  Port=2  Side=Left
  wires:
  PS-Simulink Converter/1 -> Relay/1
  PS-Simulink Converter4/1 -> Scope3/1
  Relay/1 -> Simulink-PS Converter/1, Scope/1
  connections:
  PS-Simulink Converter/LConn1 -- T input/RConn1
  DC Motor/LConn1 -- Switch/LConn1
  Switch/RConn2 -- H-Bridge/RConn1
  Controlled PWM Voltage/RConn1 -- H-Bridge/LConn1
  Ideal Rotational Motion Sensor/RConn1 -- DC Motor/RConn2 -- Mechanical Rotational Reference/LConn1
  Ideal Rotational Motion Sensor/RConn2 -- PS-Simulink Converter4/LConn1
  Ideal Rotational Motion Sensor/LConn1 -- ON/OFF FAN/RConn1 -- Gear Box/RConn1
  Controlled PWM Voltage/LConn1 -- DC Voltage Source1/LConn1
  Gear Box/LConn1 -- DC Motor/LConn2
  Electrical Reference/LConn1 -- DC Motor/RConn1 -- H-Bridge/RConn2 -- H-Bridge/LConn4 -- Controlled PWM Voltage/RConn2 -- H-Bridge/LConn2 -- H-Bridge/LConn3 -- Controlled PWM Voltage/LConn2 -- DC Voltage Source1/RConn1
  Switch/RConn1 -- Simulink-PS Converter/RConn1

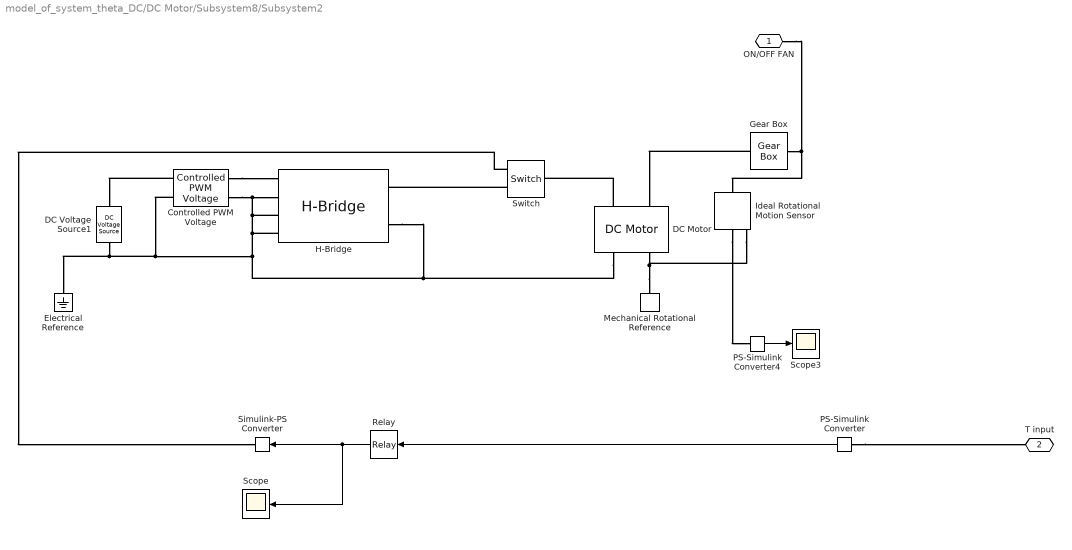
== system model_of_system_theta_DC/DC Motor/Subsystem8/Subsystem2 ==
  Controlled PWM Voltage : ee_lib/Integrated Circuits/Controlled PWM Voltage  F=4000 Hz  TD=0 s  pulse_width_offset=0 s  pulse_min=0 s  Vmin=0 V  Vmax=5 V  Vm=5 V  pwm_or_av=2  event_type=1  sample_time=1e-6 s  u_min=0  u_max=1
  DC Motor : ee_lib/Electromechanical/Brushed Motors/DC Motor  field_option=ee.enum.field_option.pm  Rf=100 Ohm  Lf=1 H  Laf=0.15 H  If0=0 A  parameterization=ee.enum.dcparam_option.load_speed  Ra=3.9 Ohm  La=.01 H  emf_or_torque=ee.enum.emf_or_torque.kv  Kv=0.072e-3 V/rpm  Ki=6.876e-4 N*m/A  T_stall=0.24e-3 N*m  w_max=4000 rpm  w_rated=1000 rpm  P_rated=10 W  V_rated=12 V  J=0.0002 kg*m^2  lam_param=ee.enum.lam_param.damping  lam=0.5e-5 N*m/(rad/s)  i_noload=0 A  V_i_noload=1.5 V  speed0=0 rpm  enable_fault_armature=ee.enum.faults.faultEnable.no  rev_faulted=1 / 3  G_faulted_armature=1e-5 S  fault_trigger_armature=ee.enum.faults.faultTrigger.temporal  t_fault_armature=1 s  max_permissible_current_armature=inf A  t_fail_on_current_armature=1 s  enable_fault_field=ee.enum.faults.faultEnable.no  G_faulted_field=1e-5 S  fault_trigger_field=ee.enum.faults.faultTrigger.temporal  t_fault_field=1 s  max_permissible_current_field=inf A  t_fail_on_current_field=1 s  fault_action=ee.enum.faults.faultAction.none  alpha=3.93e-3 1/K  Tmeas=25 degC  thermal_mass=100 J/K  initial_temperature=25 degC
  DC Voltage Source1 : fl_lib/Electrical/Electrical Sources/DC Voltage Source  v0=2.5 V
  Electrical Reference : fl_lib/Electrical/Electrical Elements/Electrical Reference
  Gear Box : fl_lib/Mechanical/Mechanisms/Gear Box  ratio=10  t_in_specify=off  t_in_priority=None  t_in=0 N*m  t_in_nominal_specify=off  t_in_nominal_unit=N*m  t_in_nominal_value=1  t_out_specify=off  t_out_priority=None  t_out=0 N*m  t_out_nominal_specify=off  t_out_nominal_unit=N*m  t_out_nominal_value=1
  H-Bridge : ee_lib/Semiconductors & Converters/Converters/H-Bridge  supply_ports=ee.enum.supply_ports.hidesupply  Venable=2.5 V  Vmax=5.0 V  Vreverse=2.5 V  Vbrake=2.5 V  Vm=12 V  pwm_or_av=ee.enum.pwm_or_av.averaged  regenerative_braking_mode=ee.enum.converters.regenerative_braking_mode.depends_on_rev  discontinuous=ee.enum.current_profile.continuous  freewheeling_mode=ee.enum.converters.freewheeling_mode.one_switch_one_diode  Ron=0.1 Ohm  Don=0.05 Ohm  Goff=1e-6 S  Rload=10 Ohm  Lload=1e-5 H  F=10 kHz  thermal_mass=100 J/K  initial_temperature=298.15 K  Ron2=0.1 Ohm  Don2=0.05 Ohm  Tmeas=298.15 K  Tmeas2=398.15 K
  Ideal Rotational Motion Sensor : fl_lib/Mechanical/Mechanical Sensors/Ideal Rotational Motion Sensor  wrap_angle=simscape.enum.onoff.off  offset=0 deg
  Mechanical Rotational Reference : fl_lib/Mechanical/Rotational Elements/Mechanical Rotational Reference
  PS-Simulink Converter : nesl_utility/PS-Simulink Converter  PhysicalDomain=network_engine_domain  SubClassName=ps_output  LeftPortType=input  RightPortType=output  PseudoPeriodic=off  Frequencies=[]  Unit=inherit  AffineConversion=off
      settings: SourceProductBaseCode=PW,SS
  PS-Simulink Converter4 : nesl_utility/PS-Simulink Converter  PhysicalDomain=network_engine_domain  SubClassName=ps_output  LeftPortType=input  RightPortType=output  PseudoPeriodic=off  Frequencies=[]  Unit=rpm  AffineConversion=off
      settings: SourceProductBaseCode=PW,SS
  Relay : Relay  OnSwitchValue=298  OffSwitchValue=295
  Scope : Scope
  Scope3 : Scope
  Simulink-PS Converter : nesl_utility/Simulink-PS Converter  PhysicalDomain=network_engine_domain  SubClassName=ps_input  LeftPortType=input  RightPortType=output  PseudoPeriodic=off  Frequencies=[]  NoiseDistribution=none  NoiseParameters=[]  Unit=1  AffineConversion=off  FilteringAndDerivatives=provide  SimscapeFilterOrder=1  InputFilterTimeConstant=0.001  UdotUserProvided=0
      settings: SourceProductBaseCode=PW,SS
  Switch : fl_lib/Electrical/Electrical Elements/Switch  R_closed=0.01 Ohm  G_open=1e-8 1/Ohm  Threshold=0.5  i_specify=off  i_priority=None  i=0 A  i_nominal_specify=off  i_nominal_unit=A  i_nominal_value=1  v_specify=off  v_priority=None  v=0 V  v_nominal_specify=off  v_nominal_unit=V  v_nominal_value=1
  ON/OFF FAN : PMIOPort  Side=Left
  T input : PMIOPort  Port=2  Side=Left
  wires:
  Relay/1 -> Scope/1, Simulink-PS Converter/1
  PS-Simulink Converter4/1 -> Scope3/1
  PS-Simulink Converter/1 -> Relay/1
  connections:
  Switch/RConn1 -- Simulink-PS Converter/RConn1
  DC Voltage Source1/RConn1 -- Controlled PWM Voltage/LConn2 -- H-Bridge/LConn3 -- H-Bridge/LConn2 -- Controlled PWM Voltage/RConn2 -- H-Bridge/LConn4 -- H-Bridge/RConn2 -- DC Motor/RConn1 -- Electrical Reference/LConn1
  Gear Box/LConn1 -- DC Motor/LConn2
  Controlled PWM Voltage/LConn1 -- DC Voltage Source1/LConn1
  Gear Box/RConn1 -- ON/OFF FAN/RConn1 -- Ideal Rotational Motion Sensor/LConn1
  Ideal Rotational Motion Sensor/RConn2 -- PS-Simulink Converter4/LConn1
  Mechanical Rotational Reference/LConn1 -- DC Motor/RConn2 -- Ideal Rotational Motion Sensor/RConn1
  Controlled PWM Voltage/RConn1 -- H-Bridge/LConn1
  Switch/RConn2 -- H-Bridge/RConn1
  DC Motor/LConn1 -- Switch/LConn1
  PS-Simulink Converter/LConn1 -- T input/RConn1
